simulink model "HybridPowertrain_TestBench_Final"  (R2017a)
settings: Solver=ode1  StartTime=0.0  StopTime=1400  FixedStep=0.01  RelTol=1e-3  EnableMultiTasking=on
undefined symbols (not defined in the file): AccActPos, air, Atm_temp, bms_inletair_temp, BMS_IstStrom, bms_maxchargecurrent, bms_maxdischargecurrent, BMS_Notfallkuehlung, BMS_SOC, BrkPdlPos, cal, Cells, Chg, D1_Commanded_Torque, D1_DC_Bus_Voltage, D2_Motor_Speed, D2_Torque_Feedback, DriverControls, EcoCAR3_Lib, Em, EngActStdyStTorq, Engine, EngSpd, env, ESS, fd, g, gb, Gearbox, GearBox, gps_lat, gps_long, Grade, I_loss, IMG, InstFuelConsmpRate, KeyPosition, lib_ESS_plant_V1_2, Loss, max_vehicle_rad_air_flow, mot, mph2kph, mph2ms, NeutralGear, ParkGear, PPEI_Engine_General_Status_2__ThrPos, PTEI_Engine_Torque_Status__EngActStdyStTorq, R_0, R_1, Ratio, RegenBrkDisable, rho, SampleTime, ShiftLeverPosition, SOC_bp, SOC_init, Spd, Speed, SW_CS_ON, SW_Engine_ON ... (+15)
libraries: simulink x39, fl_lib x13, nesl_utility x8, Utility x1, EC2_libraries x1
(part 2 of 5)

== system HybridPowertrain_TestBench_Final/ESS/ESS ==
  note: Sensors
  note: Discharge is Negative!
  note: $Author: eo1000 $
      | $Rev: 431 $
      | $Date: 2016-09-24 14:28:33 -0500 (Sat, 24 Sep 2016) $
  "In " : Inport
  "Crr " : Inport  Port=2
  0 current : Memory  InheritSampleTime=on
  Bosch_Li_Cell : Subsystem
  Bus Creator1 : BusCreator  Inputs=5
  Constant{1..4} (4 alike) : Constant  Value=0
  Cooling_Loop : Subsystem
  Cooling_Loop1 : Subsystem  Commented=on
  Data Type Conversion : DataTypeConversion  OutDataTypeStr=double
  Fault_Insertion : Subsystem
  Gain1 : Gain  Gain=Cells*0.9824
  Rate Transition : RateTransition  X0=273.15+25
  Switch1 : Switch  Threshold=1
  Switch2 : Switch  Threshold=1
  Switch3 : Switch  Threshold=5
  Switch4 : Switch  Threshold=5
  To Workspace1 : ToWorkspace  VariableName=SOC  SampleTime=-1
      settings: Decimation=WORKSPACE_DECIMATION
  To Workspace4 : ToWorkspace  VariableName=ess_current_hist  SampleTime=-1
      settings: Decimation=WORKSPACE_DECIMATION
  To Workspace5 : ToWorkspace  VariableName=ess_term_voltage_hist  SampleTime=-1
      settings: Decimation=WORKSPACE_DECIMATION
  To Workspace6 : ToWorkspace  VariableName=ess_mainc_hist  SampleTime=-1
      settings: Decimation=WORKSPACE_DECIMATION
  tloop2 : Gain  Gain=-1
  out : Outport
  Voltage : Outport  Port=2
  tag scope: SOC=global, ess_temp=global
  wires:
  "In "/1 -> [ess_mainc_stat]
  Bus Creator1/1 -> out/1
  Data Type Conversion/1 -> To Workspace6/1
  Constant2/1 -> Switch1/3
  Switch1/1 -> To Workspace4/1  "ess_ibat"
  Gain1/1 -> Switch2/1  "output voltage"
  [ess_mainc_stat] -> Switch3/2, Data Type Conversion/1, Switch3/3  "MainC"
  Constant3/1 -> Switch2/3
  Switch2/1 -> Bus Creator1/1, Voltage/1, To Workspace5/1  "ess_vbat"
  [SOC] -> Bus Creator1/5  "ess_soc"
  Bosch_Li_Cell/1(V) -> Bus Creator1/3, Gain1/1  "Vcell"
  Constant1/1 -> Switch3/1
  Switch3/1 -> Switch1/2
  [ess_mainc_stat] -> Switch4/3, Switch4/2  "MainC"
  Constant4/1 -> Switch4/1
  Switch4/1 -> Switch2/2
  0 current/1 -> tloop2/1, Bus Creator1/4, Switch1/1  "ess_ibat"
  "Crr "/1 -> 0 current/1  "current"
  Bosch_Li_Cell/3(T) -> Rate Transition/1  "T"
  Bosch_Li_Cell/2(SOC) -> To Workspace1/1, [SOC]  "SOC"
  tloop2/1 -> Bosch_Li_Cell/1(I)
  Fault_Insertion/1(Out1) -> Bus Creator1/2, [ess_temp]
  Rate Transition/1 -> Fault_Insertion/1(In1)
  connections:
  Cooling_Loop/RConn1 -- Bosch_Li_Cell/LConn1

== system HybridPowertrain_TestBench_Final/ESS/Inputs ==
  Bus Creator1 : BusCreator  Inputs=2
  CAN_fromHCU : Subsystem
  Digital_fromHCU : Subsystem
  Inputs : Outport
  wires:
  Digital_fromHCU/1(Outputs) -> Bus Creator1/2  "Digital"
  CAN_fromHCU/1(Outputs) -> Bus Creator1/1  "CAN"
  Bus Creator1/1 -> Inputs/1

== system HybridPowertrain_TestBench_Final/ESS/Outputs ==
  Outputs : Inport
  tag scope: BMS_to_HCU=global
  wires:
  Outputs/1 -> [BMS_to_HCU]  "BMS_CAN"

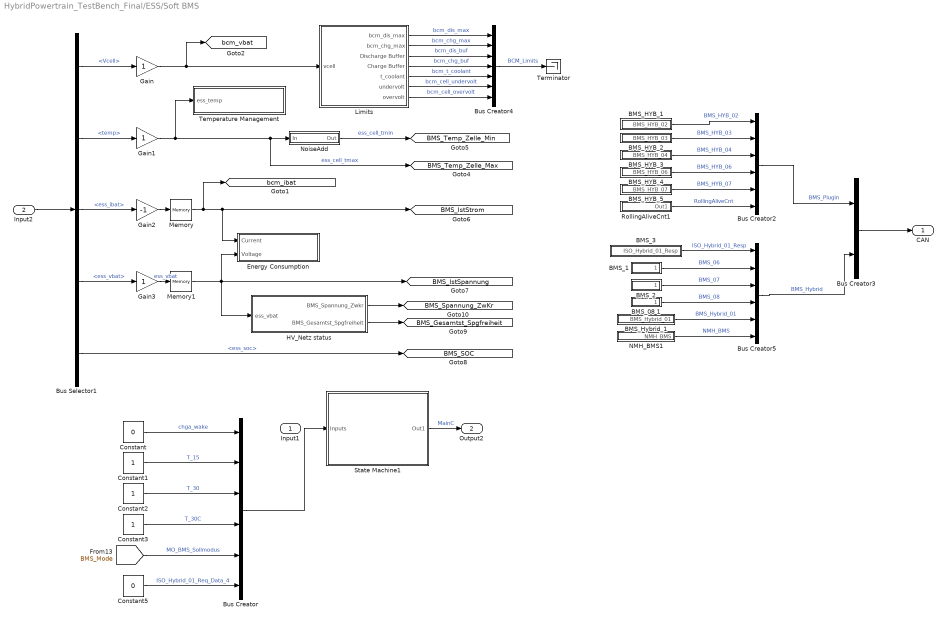
== system HybridPowertrain_TestBench_Final/ESS/Soft BMS ==
  Input1 : Inport
  Input2 : Inport  Port=2
  BMS_08 1 : Subsystem
  BMS_1 : Subsystem
  BMS_2 : Subsystem
  BMS_3 : Subsystem
  BMS_HYB_1 : Subsystem
  BMS_HYB_2 : Subsystem
  BMS_HYB_3 : Subsystem
  BMS_HYB_4 : Subsystem
  BMS_HYB_5 : Subsystem
  BMS_Hybrid_1 : Subsystem
  Bus Creator : BusCreator  Inputs=6
  Bus Creator2 : BusCreator  Inputs=6
  Bus Creator3 : BusCreator  Inputs=2
  Bus Creator4 : BusCreator  Inputs=7
  Bus Creator5 : BusCreator  Inputs=6
  Bus Selector1 : BusSelector  OutputSignals=Vcell,temp,ess_ibat,ess_vbat,ess_soc
  Constant : Constant  Value=0
  Constant1 : Constant
  Constant2 : Constant
  Constant3 : Constant
  Constant5 : Constant  Value=0
  Energy Consumption : Subsystem
  Gain : Gain
  Gain1 : Gain
  Gain2 : Gain  Gain=-1
  Gain3 : Gain
  HV_Netz status : Subsystem
  Limits : Subsystem
  Memory : Memory
  Memory1 : Memory
  NMH_BMS1 : Subsystem
  NoiseAdd : Subsystem
  RollingAliveCnt1 : Subsystem
  State Machine1 : Subsystem
  Temperature Management : Subsystem
  Terminator : Terminator
  CAN : Outport
  Output2 : Outport  Port=2
  tag scope: BMS_Gesamtst_Spgfreiheit=global, BMS_IstSpannung=global, BMS_IstStrom=global, BMS_SOC=global, BMS_Spannung_ZwKr=global, BMS_Temp_Zelle_Max=global, BMS_Temp_Zelle_Min=global, bcm_ibat=global, bcm_vbat=global
  wires:
  State Machine1/1(Out1) -> Output2/1  "MainC"
  Gain3/1 -> Memory1/1  "ess_vbat"
  Gain2/1 -> Memory/1
  Gain/1 -> [bcm_vbat], Limits/1(vcell)
  Bus Creator/1 -> State Machine1/1(Inputs)
  Input2/1 -> Bus Selector1/1
  Bus Selector1/3 -> Gain2/1  "<ess_ibat>"
  NoiseAdd/1(Out) -> [BMS_Temp_Zelle_Min]  "ess_cell_tmin"
  Bus Selector1/1 -> Gain/1  "<Vcell>"
  Bus Selector1/2 -> Gain1/1  "<temp>"
  Gain1/1 -> Temperature Management/1(ess_temp), NoiseAdd/1(In), [BMS_Temp_Zelle_Max]  "ess_cell_tmax"
  Limits/1(bcm_dis_max) -> Bus Creator4/1  "bcm_dis_max"
  Limits/3(Discharge Buffer) -> Bus Creator4/3  "bcm_dis_buf"
  Limits/4(Charge Buffer) -> Bus Creator4/4  "bcm_chg_buf"
  Limits/5(t_coolant) -> Bus Creator4/5  "bcm_t_coolant"
  Limits/2(bcm_chg_max) -> Bus Creator4/2  "bcm_chg_max"
  Bus Creator4/1 -> Terminator/1  "BCM_Limits"
  Bus Selector1/5 -> [BMS_SOC]  "<ess_soc>"
  Bus Selector1/4 -> Gain3/1  "<ess_vbat>"
  Limits/6(undervolt) -> Bus Creator4/6  "bcm_cell_undervolt"
  Limits/7(overvolt) -> Bus Creator4/7  "bcm_cell_overvolt"
  Bus Creator3/1 -> CAN/1
  HV_Netz status/1(BMS_Spannung_Zwkr) -> [BMS_Spannung_ZwKr]
  HV_Netz status/2(BMS_Gesamtst_Spgfreiheit) -> [BMS_Gesamtst_Spgfreiheit]
  Memory/1 -> [bcm_ibat], Energy Consumption/1(Current), [BMS_IstStrom]
  Memory1/1 -> [BMS_IstSpannung], HV_Netz status/1(ess_vbat), Energy Consumption/2(Voltage)
  NMH_BMS1/1(NMH_BMS) -> Bus Creator5/6  "NMH_BMS"
  BMS_HYB_2/1(BMS_HYB_03) -> Bus Creator2/2  "BMS_HYB_03"
  BMS_HYB_5/1(BMS_HYB_07) -> Bus Creator2/5  "BMS_HYB_07"
  BMS_Hybrid_1/1(BMS_Hybrid_01) -> Bus Creator5/5  "BMS_Hybrid_01"
  BMS_2/1(BMS_07) -> Bus Creator5/3  "BMS_07"
  BMS_HYB_3/1(BMS_HYB_04) -> Bus Creator2/3  "BMS_HYB_04"
  BMS_HYB_1/1(BMS_HYB_02) -> Bus Creator2/1  "BMS_HYB_02"
  BMS_HYB_4/1(BMS_HYB_06) -> Bus Creator2/4  "BMS_HYB_06"
  BMS_1/1(BMS_06) -> Bus Creator5/2  "BMS_06"
  BMS_08 1/1(BMS_08) -> Bus Creator5/4  "BMS_08"
  Bus Creator5/1 -> Bus Creator3/2  "BMS_Hybrid"
  Bus Creator2/1 -> Bus Creator3/1  "BMS_Plugin"
  BMS_3/1(ISO_Hybrid_01_Resp) -> Bus Creator5/1  "ISO_Hybrid_01_Resp"
  RollingAliveCnt1/1(Out1) -> Bus Creator2/6  "RollingAliveCnt"
  Constant/1 -> Bus Creator/1  "chga_wake"
  Constant1/1 -> Bus Creator/2  "T_15"
  Constant3/1 -> Bus Creator/4  "T_30C"
  Constant2/1 -> Bus Creator/3  "T_30"
  [BMS_Mode] -> Bus Creator/5  "MO_BMS_Sollmodus"
  Constant5/1 -> Bus Creator/6  "ISO_Hybrid_01_Req_Data_4"

== system HybridPowertrain_TestBench_Final/ICE Simple/Engine Plant Modified ==
  "In " : Inport
  eng_spd_out : Inport  Port=2
  Core Engine : Subsystem
      mask Display: image(imread('EngineShortBlock.jpg'),'center')
  ECU Actuators : Subsystem
  ECU Sensors : Subsystem
  Fuel Supply : Subsystem
      mask Display: image(imread('FuelTank.jpg'),'center')
  Radiator : Subsystem  Commented=on  AncestorBlock=lib_Vehicle/Vehicle_Plant_Model/Radiator
  Out : Outport
  eng_shaft_out : Outport  Port=2
  tag scope: EngCrankCmd=global, EngRunAtv=global, EngShutdown=global, Eng_Fan=global, Eng_Temp=global, FuelPumpEnable=global, ThrPstCmd_pct=global, VehSpdAvgDrvn_Eng=global
  wires:
  ECU Actuators/5(Out5) -> [EngShutdown]
  [FuelLevelPct] -> ECU Sensors/4(In4)  "FuelLevelPct"
  [EmsHC] -> ECU Sensors/6(In6)  "HC_g/s"
  [EngPe] -> ECU Sensors/5(In5)  "PE_0_1"
  [EmsCO] -> ECU Sensors/7(In7)  "CO_g/s"
  [EmsCO2] -> ECU Sensors/8(In8)  "CO2_g/s"
  [EmsNOx] -> ECU Sensors/9(In9)  "NOx_g/s"
  Fuel Supply/1(Available Fuel) -> Core Engine/2(Available Fuel)
  ECU Actuators/4(Out4) -> [FuelPumpEnable]
  ECU Actuators/1(Out1) -> [ThrPstCmd_pct]
  "In "/1 -> ECU Actuators/1(In1)
  [EngBrkTrq] -> ECU Sensors/1(In1)  "EngActStdyStTorq_Nm"
  [AdvFuelFlowEst] -> ECU Sensors/3(In3)  "EngFuelFlow_g/s"
  [EngSpd_RPM] -> ECU Sensors/2(In2)  "EngSpd_RPM"
  ECU Actuators/2(Out2) -> [EngCrankCmd]
  ECU Actuators/3(Out3) -> [EngRunAtv]
  Core Engine/1(eng_shaft_out) -> eng_shaft_out/1
  eng_spd_out/1 -> Core Engine/1(Engine Speed (rad/s))
  [EngTemp] -> ECU Sensors/10(In10)  "Eng_Temp"
  [Eng_Fan] -> Radiator/2(Fans)
  [Eng_Temp] -> Radiator/1(EngCltTmp)
  ECU Actuators/6(Out6) -> [Eng_Temp]
  ECU Actuators/7(Out7) -> [Eng_Fan]
  ECU Actuators/8(Out8) -> [VehSpdAvgDrvn_Eng]
  ECU Sensors/1(Out1) -> Out/1

== system HybridPowertrain_TestBench_Final/ICE Simple/Inputs ==
  Analog : Subsystem
  Bus Creator : BusCreator  Inputs=2
  CAN_from_HCU : Subsystem
  Inputs : Outport
  wires:
  CAN_from_HCU/1(Out1) -> Bus Creator/1  "CAN"
  Analog/1(Out1) -> Bus Creator/2  "Analog"
  Bus Creator/1 -> Inputs/1

== system HybridPowertrain_TestBench_Final/ICE Simple/Soft ECM ==
  note: Should check lookup table with GM
  In : Inport
  In1 : Inport  Port=2
  Bus Creator1 : BusCreator  Inputs=3
  Bus Creator2 : BusCreator  Inputs=9
  Bus Selector : BusSelector  OutputSignals=EngSpd_RPM
  Bus Selector1 : BusSelector  Commented=on  OutputSignals=Analog.EngAppReq,CAN.to EBCAN.ISO_Hybrid_01_Req.ISO_Hybrid_01_Req_Data_4,CAN.to EBCAN.PPEI_Trans_General_Status_2.TrnsShftLvrPos
  Bus Selector2 : BusSelector  OutputSignals=Eng_Temp,EngFuelFlow_g/s
  Bus Selector3 : BusSelector  OutputSignals=drv_APP1,KeyPos,ShiftLvrPos
  Data Type Conversion : DataTypeConversion  OutDataTypeStr=int8
  Data Type Conversion1 : DataTypeConversion  OutDataTypeStr=int8
  ECM_RollingAliveCnt : Subsystem
  Fuel Consumption : Subsystem
  Logic : Stateflow chart  TreatAsAtomicUnit=on
  Memory1 : Memory  X0=Engine.Init_T_amb
  Memory2 : Memory  InheritSampleTime=on
  temp vs fan : Lookup_n-D  NumberOfTableDimensions=1  BreakpointsForDimension1=[0:1:100]  Table=[0:0.01:1]  InternalRulePriority=Speed  RndMeth=Simplest  InputSameDT=on
  Out : Outport
  Out1 : Outport  Port=2
  wires:
  Logic/3(EngRunAtv) -> Bus Creator2/3  "EngRunAtv"
  Bus Selector/1 -> Logic/4(EngSpd_RPM)  "<EngSpd_RPM>"
  Bus Selector3/1 -> Memory2/1  "<drv_APP1>"
  Logic/2(EngCrankCmd) -> Bus Creator2/2  "Eng12vStrtrMtrCmmdOn"
  Bus Creator1/1 -> Out/1  "ECM_CAN"
  Bus Creator2/1 -> Out1/1, Bus Creator1/1  "ECM_to_Actuators"
  Logic/1(ThrottleCmd) -> Bus Creator2/1  "ThrPosCmd_%"
  In1/1 -> Bus Selector2/1, Bus Creator1/3, Bus Selector/1  "Sensors_to_ECM"
  In/1 -> Bus Selector1/1  "HCU_to_ECM"
  Logic/4(FuelPumpEnable) -> Bus Creator2/4  "FuelPumpEnable"
  Bus Selector3/2 -> Data Type Conversion/1  "<KeyPos>"
  [VehSpdAvgDrvn] -> Bus Creator2/6, Logic/5(VehSpdAvgDrvn)  "VehSpdAvgDrvn"
  Bus Selector3/3 -> Data Type Conversion1/1  "<ShiftLvrPos>"
  Logic/5(EngShutdown) -> Bus Creator2/5  "EngShutdown"
  Bus Selector2/1 -> Memory1/1, temp vs fan/1  "<Eng_Temp>"
  Bus Selector2/2 -> Fuel Consumption/1(Fuel Consumption)  "<EngFuelFlow_g/s>"
  Fuel Consumption/1(fuel consumption) -> Bus Creator1/2  "Eng_fuel_consumption"
  temp vs fan/1 -> Bus Creator2/9  "fan_cmd"
  Memory1/1 -> Bus Creator2/8  "Eng_Temp"
  Memory2/1 -> Logic/1(drvAPP)
  ECM_RollingAliveCnt/1(Out1) -> Bus Creator2/7
  Data Type Conversion/1 -> Logic/2(SysPwrMd)
  Data Type Conversion1/1 -> Logic/3(ShftLvrPos)
  [Driver_Request2] -> Bus Selector3/1

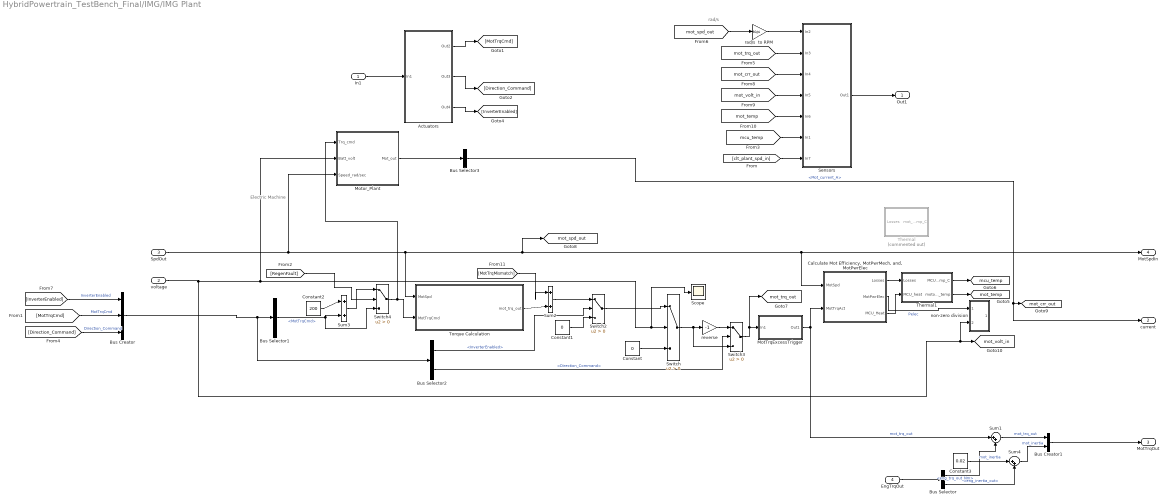
== system HybridPowertrain_TestBench_Final/IMG/IMG Plant ==
  note: Electric Machine
  note: rad/s
  "In1 " : Inport
  voltage : Inport  Port=2
  SpdOut : Inport  Port=3
  EngTrqOut : Inport  Port=4
  " Actuators" : Subsystem
  Bus Creator : BusCreator  Inputs=3
  Bus Creator1 : BusCreator  Inputs=2
  Bus Selector : BusSelector  OutputSignals=eng_trq_out_Nm,eng_inertia_out
  Bus Selector1 : BusSelector  OutputSignals=MotTrqCmd
  Bus Selector2 : BusSelector  OutputSignals=InverterEnabled,Direction_Command
  Bus Selector3 : BusSelector  OutputSignals=Mot_current_A
  "Calculate Mot Efficiency, MotPwrMech, and, MotPwrElec" : Subsystem
  Constant : Constant  Value=0
  Constant1 : Constant  Value=0
  Constant2 : Constant  Value=200
  Constant3 : Constant  Value=0.02
  MotTrqExcessTrigger : Subsystem
  Motor_Plant : Subsystem
  Scope : Scope
  Sensors : Subsystem
  Sum{1..4} (4 alike) : Sum  Inputs=|++
  Switch{,2..4} (4 alike) : Switch  Criteria=u2 > Threshold
  Thermal : Subsystem  Commented=on
  Thermal1 : Subsystem
  Torque Calculation : Subsystem
  non-zero division : Subsystem
      mask Display: disp('divider \n I1/I2')
  rad/s  to RPM : Gain  Gain=30/pi
  reverse : Gain  Gain=-1
  Out1 : Outport
  current : Outport  Port=2
  MotTrqOut : Outport  Port=3
  MotSpdIn : Outport  Port=4
  tag scope: mcu_temp=global, mot_crr_out=global, mot_spd_out=global, mot_temp=global, mot_trq_out=global, mot_volt_in=global
  wires:
  [mot_temp] -> Sensors/5(In6)
  [mot_crr_out] -> Sensors/3(In4)
  "In1 "/1 -> " Actuators"/1(In1)
  [mot_volt_in] -> Sensors/4(In5)
  " Actuators"/1(Out2) -> [MotTrqCmd]
  Sensors/1(Out1) -> Out1/1
  [mot_trq_out] -> Sensors/2(In3)
  SpdOut/1 -> Motor_Plant/3(Speed_rad/sec), Torque Calculation/1(MotSpd), [mot_spd_out], MotSpdIn/1, "Calculate Mot Efficiency, MotPwrMech, and, MotPwrElec"/1(MotSpd)
  Bus Selector3/1 -> current/1, [mot_crr_out]  "<Mot_current_A>"
  [mcu_temp] -> Sensors/6(In1)
  [clt_plant_spd_in] -> Sensors/7(In7)
  " Actuators"/2(Out3) -> [Direction_Command]
  " Actuators"/3(Out4) -> [InverterEnabled]
  [Direction_Command] -> Bus Creator/3  "Direction_Command"
  [InverterEnabled] -> Bus Creator/1  "InverterEnabled"
  [MotTrqCmd] -> Bus Creator/2  "MotTrqCmd"
  [mot_spd_out] -> rad/s  to RPM/1
  rad/s  to RPM/1 -> Sensors/1(In2)
  Thermal1/1(MCU_temp_C) -> [mcu_temp]
  Constant2/1 -> Sum3/1
  Switch4/1 -> Motor_Plant/1(Trq_cmd), Torque Calculation/2(MotTrqCmd)
  Sum3/1 -> Switch4/1
  [RegenFault] -> Switch4/2
  Switch3/1 -> [mot_trq_out], MotTrqExcessTrigger/1(In1)
  reverse/1 -> Switch3/1
  Bus Selector2/2 -> Switch3/2  "<Direction_Command>"
  Switch2/1 -> Switch/1
  Constant1/1 -> Switch2/3
  Bus Selector2/1 -> Switch2/2  "<InverterEnabled>"
  Bus Selector1/1 -> Switch4/3, Sum3/2  "<MotTrqCmd>"
  Bus Creator/1 -> Bus Selector2/1, Bus Selector1/1
  Sum2/1 -> Switch2/1
  Torque Calculation/1(mot_trq_out) -> Sum2/2
  [MotTrqMismatch] -> Sum2/1
  Switch/1 -> Switch3/3, reverse/1
  Thermal1/2(motor_temp) -> [mot_temp]
  "Calculate Mot Efficiency, MotPwrMech, and, MotPwrElec"/3(MCU_Heat) -> Thermal1/2(MCU_heat)
  Constant/1 -> Switch/3
  "Calculate Mot Efficiency, MotPwrMech, and, MotPwrElec"/1(Losses) -> Thermal1/1(Losses)
  MotTrqExcessTrigger/1(Out1) -> Sum1/1, "Calculate Mot Efficiency, MotPwrMech, and, MotPwrElec"/2(MotTrqAct)  "mot_trq_out"
  "Calculate Mot Efficiency, MotPwrMech, and, MotPwrElec"/2(MotPwrElec) -> non-zero division/1(In1)  "Pelec"
  voltage/1 -> non-zero division/2(In2), [mot_volt_in], Motor_Plant/2(Batt_volt), Scope/1, Switch/2
  Bus Creator1/1 -> MotTrqOut/1
  Sum4/1 -> Bus Creator1/2  "mot_inertia"
  EngTrqOut/1 -> Bus Selector/1
  Sum1/1 -> Bus Creator1/1  "mot_trq_out"
  Bus Selector/2 -> Sum4/2  "<eng_inertia_out>"
  Constant3/1 -> Sum4/1  "mot_inertia"
  Bus Selector/1 -> Sum1/2  "<eng_trq_out_Nm>"
  Motor_Plant/1(Mot_out) -> Bus Selector3/1

== system HybridPowertrain_TestBench_Final/IMG/Soft MCU ==
  In : Inport
  In1 : Inport  Port=2
  Bus Creator : BusCreator  Inputs=6
  Bus Creator1 : BusCreator  Inputs=2
  Bus Selector : BusSelector  OutputSignals=mot_spd_out,mot_trq_out
  Bus Selector1 : BusSelector  Commented=on  OutputSignals=M192_Command_Message.Inverter_Enable,M192_Command_Message.Torque_Command
  Constant : Constant  Value=0
  Constant1 : Constant
  Data Type Conversion{1..4} (4 alike) : DataTypeConversion
  ForwardDirection : Constant  Value=0
  MCU_CAN_rolling : Subsystem
  Memory : Memory
  Scope : Scope  NumInputPorts=5
  Switch : Switch  Threshold=1
  Torque Calculation : Subsystem
  Out : Outport
  Out1 : Outport  Port=2
  wires:
  In1/1 -> Bus Creator1/2, Bus Selector/1  "Sensors_to_MCU"
  Bus Creator1/1 -> Out/1  "MCU_CAN"
  In/1 -> Bus Selector1/1  "HCU_to_MCU"
  [MotTrqCmd] -> Torque Calculation/1(MotTrqReq), Scope/2, Data Type Conversion4/1
  Bus Creator/1 -> Bus Creator1/1, Out1/1  "MCU_to _Actuator"
  Constant1/1 -> Memory/1, Switch/2, Scope/3
  Constant/1 -> Switch/3
  Bus Selector/1 -> Scope/5, Torque Calculation/2(MotSpd)  "<mot_spd_out>"
  Torque Calculation/1(mot_trq_out) -> Switch/1
  Data Type Conversion1/1 -> Bus Creator/3  "InverterEnabled"
  Bus Selector/2 -> Scope/4, Torque Calculation/3(MotTrqFdbck), Data Type Conversion2/1  "<mot_trq_out>"
  Data Type Conversion2/1 -> Bus Creator/4  "MotTrqFdbck"
  Memory/1 -> Data Type Conversion1/1
  Switch/1 -> Data Type Conversion3/1  "MotTrqCmd"
  Data Type Conversion3/1 -> Bus Creator/2, Scope/1  "MotTrqCmd"
  Data Type Conversion4/1 -> Bus Creator/1  "Torque_Command"
  MCU_CAN_rolling/1(Out1) -> Bus Creator/5  "D3_Power_On_Timer"
  ForwardDirection/1 -> Bus Creator/6  "Direction_Command"

== system HybridPowertrain_TestBench_Final/Measurements_hybrid/DriverControls1 ==
  cmd : Inport
  meas : Inport  Port=2
  BrakeForce : Gain  Gain=100
  Memory : Memory
  Memory1 : Memory
  PID Controller : simulink/Continuous/PID Controller  Controller=PI  TimeDomain=Continuous-time  SampleTime=-1  IntegratorMethod=Forward Euler  FilterMethod=Forward Euler  Form=Parallel  UseFilter=on  ControllerParametersSource=internal  P=0.1  I=0.001  D=0  N=100  InitialConditionSource=internal  InitialConditionForIntegrator=0  InitialConditionForFilter=0  ExternalReset=none  LimitOutput=off  UpperSaturationLimit=1  LowerSaturationLimit=0  LinearizeAsGain=on  AntiWindupMode=clamping  Kb=1  TrackingMode=off  Kt=1  PParamMin=[]  PParamMax=[]  IParamMin=[]  IParamMax=[]  DParamMin=[]  DParamMax=[]  NParamMin=[]  NParamMax=[]  KbParamMin=[]  KbParamMax=[]  KtParamMin=[]  KtParamMax=[]  POutMin=[]  POutMax=[]  IOutMin=[]  IOutMax=[]  DOutMin=[]  DOutMax=[]  NOutMin=[]  NOutMax=[]  KbOutMin=[]  KbOutMax=[]  KtOutMin=[]  KtOutMax=[]  IntegratorOutMin=[]  IntegratorOutMax=[]  FilterOutMin=[]  FilterOutMax=[]  SumOutMin=[]  SumOutMax=[]  SumI1OutMin=[]  SumI1OutMax=[]  SumI2OutMin=[]  SumI2OutMax=[]  SumI3OutMin=[]  SumI3OutMax=[]  SumDOutMin=[]  SumDOutMax=[]  SaturationOutMin=[]  SaturationOutMax=[]  IntegratorContinuousStateAttributes=''  IntegratorStateMustResolveToSignalObject=off  IntegratorRTWStateStorageClass=Auto  FilterContinuousStateAttributes=''  FilterStateMustResolveToSignalObject=off  FilterRTWStateStorageClass=Auto  DifferentiatorICPrevScaledInput=0  DifferentiatorOutMin=[]  DifferentiatorOutMax=[]  InitialConditionSetting=State (most efficient)
  PID Controller1 : simulink/Continuous/PID Controller  Controller=PI  TimeDomain=Continuous-time  SampleTime=-1  IntegratorMethod=Forward Euler  FilterMethod=Forward Euler  Form=Parallel  UseFilter=on  ControllerParametersSource=internal  P=0.1  I=0.001  D=0  N=100  InitialConditionSource=internal  InitialConditionForIntegrator=0  InitialConditionForFilter=0  ExternalReset=none  LimitOutput=on  UpperSaturationLimit=1  LowerSaturationLimit=-1  LinearizeAsGain=on  AntiWindupMode=clamping  Kb=1  TrackingMode=off  Kt=1  PParamMin=[]  PParamMax=[]  IParamMin=[]  IParamMax=[]  DParamMin=[]  DParamMax=[]  NParamMin=[]  NParamMax=[]  KbParamMin=[]  KbParamMax=[]  KtParamMin=[]  KtParamMax=[]  POutMin=[]  POutMax=[]  IOutMin=[]  IOutMax=[]  DOutMin=[]  DOutMax=[]  NOutMin=[]  NOutMax=[]  KbOutMin=[]  KbOutMax=[]  KtOutMin=[]  KtOutMax=[]  IntegratorOutMin=[]  IntegratorOutMax=[]  FilterOutMin=[]  FilterOutMax=[]  SumOutMin=[]  SumOutMax=[]  SumI1OutMin=[]  SumI1OutMax=[]  SumI2OutMin=[]  SumI2OutMax=[]  SumI3OutMin=[]  SumI3OutMax=[]  SumDOutMin=[]  SumDOutMax=[]  SaturationOutMin=[]  SaturationOutMax=[]  IntegratorContinuousStateAttributes=''  IntegratorStateMustResolveToSignalObject=off  IntegratorRTWStateStorageClass=Auto  FilterContinuousStateAttributes=''  FilterStateMustResolveToSignalObject=off  FilterRTWStateStorageClass=Auto  DifferentiatorICPrevScaledInput=0  DifferentiatorOutMin=[]  DifferentiatorOutMax=[]  InitialConditionSetting=State (most efficient)
  Pct : Gain  Gain=100
  Saturation1 : Saturate  UpperLimit=100  LowerLimit=0
  Saturation2 : Saturate  UpperLimit=100  LowerLimit=0
  Sum : Sum  Inputs=|+-
  Sum1 : Sum  Inputs=+-|
  brake : Outport
  throttle : Outport  Port=2
  wires:
  cmd/1 -> Sum/1, Sum1/2
  Sum1/1 -> PID Controller/1
  meas/1 -> Sum1/1, Sum/2
  PID Controller/1 -> BrakeForce/1
  Saturation1/1 -> Memory/1
  BrakeForce/1 -> Saturation1/1
  PID Controller1/1 -> Pct/1
  Memory/1 -> brake/1
  Sum/1 -> PID Controller1/1
  Pct/1 -> Saturation2/1
  Saturation2/1 -> Memory1/1
  Memory1/1 -> throttle/1

== system HybridPowertrain_TestBench_Final/Measurements_hybrid/Subsystem ==
  In1 : Inport
  Add1 : Sum  Inputs=+++
  Add2 : Sum
  Constant1 : Constant  Value=0
  Constant2 : Constant  Value=cal.APP.Mismatch_Value+0.1
  Constant3 : Constant  Value=0
  Constant4 : Constant  Value=cal.APP2.IN_Max_SC_Prcnt+1
  Constant5 : Constant  Value=0
  Constant6 : Constant  Value=cal.APP2.IN_Max_SC_Prcnt+1
  Switch : Switch  Threshold=1
  Switch1 : Switch  Threshold=1
  Switch2 : Switch  Threshold=1
  APP1 : Outport
  APP2 : Outport  Port=2
  wires:
  Switch2/1 -> Add2/2
  Add2/1 -> APP1/1  "drv_APP1"
  [APP2_OOR_ON] -> Switch2/2
  Constant6/1 -> Switch2/1
  Constant5/1 -> Switch2/3
  In1/1 -> Add1/1, Add2/1
  Add1/1 -> APP2/1  "drv_APP2"
  Switch1/1 -> Add1/3
  [APP2_OOR_ON] -> Switch1/2
  Constant4/1 -> Switch1/1
  Constant3/1 -> Switch1/3
  Constant2/1 -> Switch/1
  Constant1/1 -> Switch/3
  Switch/1 -> Add1/2
  [Mismatch_APP_ON] -> Switch/2

== system HybridPowertrain_TestBench_Final/Measurements_stock/DriverControls ==
  cmd : Inport
  meas : Inport  Port=2
  Abs : Abs
  BrakeForce : Gain  Commented=on  Gain=100
  Clamping circuit : Subsystem  Commented=on
  Compare To Constant : simulink/Logic and Bit Operations/Compare To Constant  relop=>  const=10  OutDataTypeStr=boolean
  Compare To Constant1 : simulink/Logic and Bit Operations/Compare To Constant  relop=>  const=0  OutDataTypeStr=boolean
  Compare To Constant2 : simulink/Logic and Bit Operations/Compare To Constant  relop=<=  const=0  OutDataTypeStr=boolean
  Constant : Constant  Value=11.5
  Constant1 : Constant  Commented=on  DisableCoverage=on  Value=0  OutDataTypeStr=Inherit: Inherit via back propagation  PreserveConstantTs=on
  Constant2 : Constant  Value=0
  Constant3 : Constant  Value=0
  IntegralGain : Gain  Commented=on  Gain=0.001
  Integrator : Integrator  Commented=on
  Memory : Memory  Commented=on
  MinMax : MinMax  Function=max  Inputs=2
  PID Controller : simulink/Continuous/PID Controller  Commented=on  Controller=PI  TimeDomain=Continuous-time  SampleTime=-1  IntegratorMethod=Forward Euler  FilterMethod=Forward Euler  Form=Parallel  UseFilter=on  ControllerParametersSource=internal  P=0.1  I=0.001  D=0  N=100  InitialConditionSource=internal  InitialConditionForIntegrator=0  InitialConditionForFilter=0  ExternalReset=none  LimitOutput=off  UpperSaturationLimit=1  LowerSaturationLimit=0  LinearizeAsGain=on  AntiWindupMode=clamping  Kb=1  TrackingMode=off  Kt=1  PParamMin=[]  PParamMax=[]  IParamMin=[]  IParamMax=[]  DParamMin=[]  DParamMax=[]  NParamMin=[]  NParamMax=[]  KbParamMin=[]  KbParamMax=[]  KtParamMin=[]  KtParamMax=[]  POutMin=[]  POutMax=[]  IOutMin=[]  IOutMax=[]  DOutMin=[]  DOutMax=[]  NOutMin=[]  NOutMax=[]  KbOutMin=[]  KbOutMax=[]  KtOutMin=[]  KtOutMax=[]  IntegratorOutMin=[]  IntegratorOutMax=[]  FilterOutMin=[]  FilterOutMax=[]  SumOutMin=[]  SumOutMax=[]  SumI1OutMin=[]  SumI1OutMax=[]  SumI2OutMin=[]  SumI2OutMax=[]  SumI3OutMin=[]  SumI3OutMax=[]  SumDOutMin=[]  SumDOutMax=[]  SaturationOutMin=[]  SaturationOutMax=[]  IntegratorContinuousStateAttributes=''  IntegratorStateMustResolveToSignalObject=off  IntegratorRTWStateStorageClass=Auto  FilterContinuousStateAttributes=''  FilterStateMustResolveToSignalObject=off  FilterRTWStateStorageClass=Auto  DifferentiatorICPrevScaledInput=0  DifferentiatorOutMin=[]  DifferentiatorOutMax=[]
  PID Controller1 : simulink/Continuous/PID Controller  Controller=PI  TimeDomain=Continuous-time  SampleTime=-1  IntegratorMethod=Forward Euler  FilterMethod=Forward Euler  Form=Parallel  UseFilter=on  ControllerParametersSource=internal  P=0.1  I=0.001  D=0  N=100  InitialConditionSource=internal  InitialConditionForIntegrator=0  InitialConditionForFilter=0  ExternalReset=none  LimitOutput=on  UpperSaturationLimit=1  LowerSaturationLimit=-1  LinearizeAsGain=on  AntiWindupMode=clamping  Kb=1  TrackingMode=off  Kt=1  PParamMin=[]  PParamMax=[]  IParamMin=[]  IParamMax=[]  DParamMin=[]  DParamMax=[]  NParamMin=[]  NParamMax=[]  KbParamMin=[]  KbParamMax=[]  KtParamMin=[]  KtParamMax=[]  POutMin=[]  POutMax=[]  IOutMin=[]  IOutMax=[]  DOutMin=[]  DOutMax=[]  NOutMin=[]  NOutMax=[]  KbOutMin=[]  KbOutMax=[]  KtOutMin=[]  KtOutMax=[]  IntegratorOutMin=[]  IntegratorOutMax=[]  FilterOutMin=[]  FilterOutMax=[]  SumOutMin=[]  SumOutMax=[]  SumI1OutMin=[]  SumI1OutMax=[]  SumI2OutMin=[]  SumI2OutMax=[]  SumI3OutMin=[]  SumI3OutMax=[]  SumDOutMin=[]  SumDOutMax=[]  SaturationOutMin=[]  SaturationOutMax=[]  IntegratorContinuousStateAttributes=''  IntegratorStateMustResolveToSignalObject=off  IntegratorRTWStateStorageClass=Auto  FilterContinuousStateAttributes=''  FilterStateMustResolveToSignalObject=off  FilterRTWStateStorageClass=Auto  DifferentiatorICPrevScaledInput=0  DifferentiatorOutMin=[]  DifferentiatorOutMax=[]
  Pct : Gain  Gain=100
  ProportionalGain : Gain  Commented=on  Gain=0.1
  Saturation : Saturate  UpperLimit=100  LowerLimit=-100  LinearizeAsGain=off
  Saturation1 : Saturate  Commented=on  UpperLimit=100  LowerLimit=0
  Sum : Sum  Inputs=|+-
  Sum1 : Sum  Commented=on  Inputs=+-|
  Sum3 : Sum  Commented=on  Inputs=++|
  Switch : Switch  Criteria=u2 > Threshold
  Switch1 : Switch  Commented=on  Criteria=u2 > Threshold  SampleTime=SampleTime  InputSameDT=on
  Switch2 : Switch  Criteria=u2 > Threshold
  Switch3 : Switch  Criteria=u2 > Threshold
  brake : Outport
  throttle : Outport  Port=2
  wires:
  cmd/1 -> Compare To Constant/1, Sum/1, Sum1/2
  Sum1/1 -> PID Controller/1
  meas/1 -> Sum1/1, Sum/2
  PID Controller/1 -> BrakeForce/1
  Saturation1/1 -> Memory/1
  BrakeForce/1 -> Saturation1/1
  PID Controller1/1 -> Pct/1
  Memory/1 -> ?
  Compare To Constant/1 -> Switch/2
  MinMax/1 -> Switch/3
  Constant/1 -> MinMax/2
  Saturation/1 -> ?
  Sum/1 -> PID Controller1/1, ProportionalGain/1, IntegralGain/1
  Integrator/1 -> Sum3/2
  ProportionalGain/1 -> Sum3/1
  Sum3/1 -> Clamping circuit/1(preSat)
  Constant1/1 -> Switch1/1
  Clamping circuit/1(Clamp) -> Switch1/2
  IntegralGain/1 -> Integrator/1, Clamping circuit/2(preIntegrator), Switch1/3
  Compare To Constant1/1 -> Switch2/2
  Constant2/1 -> Switch2/3
  Switch2/1 -> throttle/1
  Pct/1 -> Compare To Constant2/1, Abs/1, Switch2/1, Compare To Constant1/1, Saturation/1, Switch/1, MinMax/1
  Compare To Constant2/1 -> Switch3/2
  Constant3/1 -> Switch3/3
  Switch3/1 -> brake/1
  Abs/1 -> Switch3/1

== system HybridPowertrain_TestBench_Final/Measurements_stock/Subsystem ==
  In1 : Inport
  Add1 : Sum  Inputs=+++
  Add2 : Sum
  Constant1 : Constant  Value=0
  Constant2 : Constant  Value=cal.APP.Mismatch_Value+0.1
  Constant3 : Constant  Value=0
  Constant4 : Constant  Value=cal.APP2.IN_Max_SC_Prcnt+1
  Constant5 : Constant  Value=0
  Constant6 : Constant  Value=cal.APP2.IN_Max_SC_Prcnt+1
  Switch : Switch  Threshold=1
  Switch1 : Switch  Threshold=1
  Switch2 : Switch  Threshold=1
  APP1 : Outport
  APP2 : Outport  Port=2
  wires:
  [Mismatch_APP_ON] -> Switch/2
  Switch/1 -> Add1/2
  Constant1/1 -> Switch/3
  Constant2/1 -> Switch/1
  Constant3/1 -> Switch1/3
  Constant4/1 -> Switch1/1
  [APP2_OOR_ON] -> Switch1/2
  Switch1/1 -> Add1/3
  Add1/1 -> APP2/1  "drv_APP2"
  In1/1 -> Add2/1, Add1/1
  Constant5/1 -> Switch2/3
  Constant6/1 -> Switch2/1
  [APP2_OOR_ON] -> Switch2/2
  Add2/1 -> APP1/1  "drv_APP1"
  Switch2/1 -> Add2/2

== system HybridPowertrain_TestBench_Final/Transmission/Inputs ==
  Analog_fromHCU : Subsystem
  Bus Creator1 : BusCreator  Inputs=3
  CAN_fromHCU : Subsystem
  Digital_fromHCU : Subsystem
  Inputs : Outport
  wires:
  Digital_fromHCU/1(Outputs) -> Bus Creator1/2  "Digital"
  CAN_fromHCU/1(Outputs) -> Bus Creator1/1  "CAN"
  Bus Creator1/1 -> Inputs/1
  Analog_fromHCU/1(Outputs) -> Bus Creator1/3

== system HybridPowertrain_TestBench_Final/Transmission/Outputs ==
  Outputs : Inport
  tag scope: TCM_to_HCU=global
  wires:
  Outputs/1 -> [TCM_to_HCU]  "TCM_CAN"

== system HybridPowertrain_TestBench_Final/Transmission/Soft TCM ==
  In : Inport
  In1 : Inport  Port=2
  6L45 Logic : Stateflow chart  TreatAsAtomicUnit=on
  Bus Creator : BusCreator  Inputs=3
  Bus Creator1 : BusCreator  Inputs=2
  Bus Selector : BusSelector  OutputSignals=impeller_spd_rads,turbine_spd_rads
  Bus Selector1 : BusSelector  Commented=on  OutputSignals=CAN.PPEI_Engine_General_Status_1.AccActPos,CAN.PPEI_Vehicle_Speed_and_Distance.VehSpdAvgDrvn
  Bus Selector2 : BusSelector  OutputSignals=drv_APP1,Veh_Spd
  Data Type Conversion : DataTypeConversion
  TorqConv Lockup threshold : Constant  Value=tc.plant.init.lock_thresh
  Out : Outport
  Out1 : Outport  Port=2
  wires:
  TorqConv Lockup threshold/1 -> 6L45 Logic/1(tc_lockup_thrsh)
  6L45 Logic/1(TransEstGear) -> Bus Creator/1
  Data Type Conversion/1 -> Bus Creator/3, 6L45 Logic/7(ShftLvrPos)  "TrnsShftLvrPos"
  In1/1 -> Bus Selector/1, Bus Creator1/2  "Sensors_to_TCM"
  Bus Creator1/1 -> Out/1  "TCM_CAN"
  In/1 -> Bus Selector1/1  "HCU_to_TCM"
  Bus Selector/2 -> 6L45 Logic/5(tc_spd_out)  "<turbine_spd_rads>"
  Bus Selector/1 -> 6L45 Logic/4(tc_spd_in)  "<impeller_spd_rads>"
  [chas_plant_lin_spd_out] -> 6L45 Logic/3(VehicleSpeed)
  Bus Selector2/1 -> 6L45 Logic/2(drvAPP)  "<drv_APP1>"
  Bus Creator/1 -> Out1/1, Bus Creator1/1  "TCM_to _Actuator"
  6L45 Logic/2(LockupCmd) -> Bus Creator/2
  [drv_BPP_percent] -> 6L45 Logic/6(drvBPP)
  [ShftLvrPos] -> Data Type Conversion/1  "TrnsShftLvrPos"
  [Driver_Request2] -> Bus Selector2/1

== system HybridPowertrain_TestBench_Final/Transmission/Transmission Plant ==
  "In1 " : Inport
  TorqConvShaftIn : Inport  Port=2
  GearboxSpdOut : Inport  Port=3
  " Actuators" : Subsystem
  Gearbox : Subsystem
      mask Display:
      | image('Images\Gearbox.jpg')
      | color('red');
      | port_label('Input',1,'Gear');
      | port_label('Input',2,'ShftIn');
      | port_label('Input',3,'SpdOut');
      | port_label('Output',1,'ShaftOut');
      | port_label('Output',2,'SpdIn');
  Sensors : Subsystem
  Torque Converter : Subsystem
      mask Display:
      | image('Images\TorqConv.jpg')
      | color('red');
      | port_label('Input',2,'ShaftIn');
      | port_label('Input',3,'SpdOut');
      | port_label('Output',1,'ShaftOut');
      | port_label('Output',2,'SpdIn');
  Out1 : Outport
  GearboxShaftOut : Outport  Port=2
  TorqConvSpdIn : Outport  Port=3
  tag scope: TransEstGear=global
  wires:
  Torque Converter/2(cpl_spd_in) -> TorqConvSpdIn/1
  Gearbox/2(gb_spd_in) -> Torque Converter/3(tc_spd_out)
  TorqConvShaftIn/1 -> Torque Converter/2(tc_shaft_in)
  Gearbox/1(gb_trq_out gb_inertia_out) -> GearboxShaftOut/1
  " Actuators"/1(Out2) -> [TransEstGear]
  [tc_trq_out] -> Sensors/4(In5)
  [gb_spd_out] -> Sensors/5(In6)
  [gb_trq_out] -> Sensors/6(In7)
  [tc_spd_out] -> Sensors/2(In3)
  [tc_spd_in] -> Sensors/1(In2)
  [tc_trq_in] -> Sensors/3(In4)
  " Actuators"/2(Out5) -> [LockupCmd]
  "In1 "/1 -> " Actuators"/1(In1)
  Sensors/1(Out1) -> Out1/1
  [TransEstGear] -> Gearbox/1(TransEstGear)
  Torque Converter/1(tc_shaft_out) -> Gearbox/2(gb_trq_in gb_inertia_in)
  GearboxSpdOut/1 -> Gearbox/3(gb_spd_out)
  [LockupCmd] -> Torque Converter/1(tc_lockup)
  [gb_trq_ratio] -> Sensors/7(In1)

== system HybridPowertrain_TestBench_Final/Wheels/Force calculation ==
  spd in : Inport
  BPP[%] : Inport  Port=2
  whl_spd : Inport  Port=3
  grade : Inport  Port=4
  trq_in : Inport  Port=5
  Inertia_In : Inport  Port=6
  "1\\radius " : Gain  Gain=1/whl.plant.init.radius  SaturateOnIntegerOverflow=on  OutDataTypeStr=Inherit: Same as input  ParamDataTypeStr=Inherit: Same as input
  1\radius 1 : Gain  Gain=-1/100  SaturateOnIntegerOverflow=on  OutDataTypeStr=Inherit: Same as input  ParamDataTypeStr=Inherit: Same as input
  Blending : Subsystem  mask(State dependent blending){xl=-0.1, yl=-1, xc=0, yc=0, xr=0.1, yr=1}
      mask prompts: xl "Left point (x-value):"; yl "Left point (y-value):"; xc "Center point (x-value):"; yc "Center point (y-value):"; xr "Right point (x-value):"; yr "Right point (y-vector):"
      mask Display: plot([-1 1 3 6 8], [1.5 1.5 0.5 4.0 4.0])
  Derivative : Derivative
  Divide : Product  Inputs=**
  Rolling Resistance : Subsystem
  Saturation1 : Saturate  UpperLimit=0  LowerLimit=-inf
  Scope : Scope
  Sum2 : Sum  Inputs=++--  SaturateOnIntegerOverflow=on  InputSameDT=on  OutDataTypeStr=Inherit: Same as first input
  Sum6 : Sum  SaturateOnIntegerOverflow=on  InputSameDT=on  OutDataTypeStr=Inherit: Same as first input
  trq_brake_max : Gain  Gain=whl.plant.init.trq_brake_max
  wheel inertia : Constant  Value=whl.plant.init.inertia
  force : Outport
  wires:
  Rolling Resistance/1(rolling resistance) -> Sum2/3
  grade/1 -> Rolling Resistance/2(grade)
  whl_spd/1 -> Rolling Resistance/1(whl_spd)
  trq_brake_max/1 -> Blending/1(input)
  Sum2/1 -> "1\\radius "/1
  Saturation1/1 -> Scope/1, Sum2/1
  BPP[%]/1 -> 1\radius 1/1  "brake cmd"
  spd in/1 -> Derivative/1, Blending/2(Control (state))
  trq_in/1 -> Sum2/2
  1\radius 1/1 -> trq_brake_max/1
  "1\\radius "/1 -> force/1
  Blending/1(Out1) -> Saturation1/1
  Inertia_In/1 -> Sum6/2
  Derivative/1 -> Divide/2
  Divide/1 -> Sum2/4
  wheel inertia/1 -> Sum6/1
  Sum6/1 -> Divide/1

== system HybridPowertrain_TestBench_Final/Wheels/Mass calculation ==
  inertia in : Inport
  1\radius^2 : Gain  Gain=1/whl.plant.init.radius^2  SaturateOnIntegerOverflow=on  OutDataTypeStr=Inherit: Same as input  ParamDataTypeStr=Inherit: Same as input
  Sum6 : Sum  SaturateOnIntegerOverflow=on  InputSameDT=on  OutDataTypeStr=Inherit: Same as first input
  wheel inertia : Constant  Value=whl.plant.init.inertia
  Mass : Outport
  wires:
  inertia in/1 -> Sum6/2
  1\radius^2/1 -> Mass/1
  Sum6/1 -> 1\radius^2/1
  wheel inertia/1 -> Sum6/1

== system HybridPowertrain_TestBench_Final/Wheels/Speed calculation ==
  chas_spd : Inport
  spd in : Outport
  wires:
  chas_spd/1 -> spd in/1

== system HybridPowertrain_TestBench_Final/Differential/Torque calculation/Blending (state dependent) ==
  Input : Inport
  Control (state) : Inport  Port=2
  Linear spline : Fcn  Expr=(u<xl)*yl + (xl<=u)*(u<xc)*((yc-yl)*(u-xl)/(xc-xl)+yl) + (xc<=u)*(u<xr)*((yc-yr)*(u-xr)/(xc-xr)+yr) + (xr<=u)*yr
  Product2 : Product  SaturateOnIntegerOverflow=on  InputSameDT=on  OutDataTypeStr=Inherit: Same as first input
  Output : Outport
  wires:
  Input/1 -> Product2/1
  Linear spline/1 -> Product2/2
  Product2/1 -> Output/1
  Control (state)/1 -> Linear spline/1

== system HybridPowertrain_TestBench_Final/Differential/Torque calculation/Look-Up Table (2-D) ==
  Rows : Inport
  Cols : Inport  Port=2
  Look-Up Table (2-D) : Lookup2D  RowIndex=x  ColumnIndex=y  Table=t  SaturateOnIntegerOverflow=on  InputSameDT=on
  Out1 : Outport
  wires:
  Rows/1 -> Look-Up Table (2-D)/1
  Cols/1 -> Look-Up Table (2-D)/2
  Look-Up Table (2-D)/1 -> Out1/1

== system HybridPowertrain_TestBench_Final/Driver/Driver Control/Override CS SW ==
  note: Override Switch Subsystem
  note: This subsystem is used to override the model value of a signal to a constant value
  In1 : Inport
  Multiport Switch : MultiPortSwitch  DataPortOrder=Zero-based contiguous  Inputs=2  zeroidx=on
  Override Value : Constant  Value=0  OutDataTypeStr=double
  Signal Override Switch 0 = Use Model 1 = Use Constant : Constant
  Out1 : Outport
  wires:
  Override Value/1 -> Multiport Switch/3
  Multiport Switch/1 -> Out1/1
  In1/1 -> Multiport Switch/2
  Signal Override Switch 0 = Use Model 1 = Use Constant/1 -> Multiport Switch/1

== system HybridPowertrain_TestBench_Final/Driver/Driver Control/Override Engine SW ==
  note: This subsystem is used to override the model value of a signal to a constant value
  note: Override Switch Subsystem
  In1 : Inport
  Multiport Switch : MultiPortSwitch  DataPortOrder=Zero-based contiguous  Inputs=2  zeroidx=on
  Override Value : Constant  Value=0  OutDataTypeStr=double
  Signal Override Switch 0 = Use Model 1 = Use Constant : Constant
  Out1 : Outport
  wires:
  Signal Override Switch 0 = Use Model 1 = Use Constant/1 -> Multiport Switch/1
  In1/1 -> Multiport Switch/2
  Multiport Switch/1 -> Out1/1
  Override Value/1 -> Multiport Switch/3

== system HybridPowertrain_TestBench_Final/Driver/Driver Control/Override Regen SW ==
  note: Override Switch Subsystem
  note: This subsystem is used to override the model value of a signal to a constant value
  In1 : Inport
  Multiport Switch : MultiPortSwitch  DataPortOrder=Zero-based contiguous  Inputs=2  zeroidx=on
  Override Value : Constant  Value=0  OutDataTypeStr=double
  Signal Override Switch 0 = Use Model 1 = Use Constant : Constant
  Out1 : Outport
  wires:
  Override Value/1 -> Multiport Switch/3
  Multiport Switch/1 -> Out1/1
  In1/1 -> Multiport Switch/2
  Signal Override Switch 0 = Use Model 1 = Use Constant/1 -> Multiport Switch/1

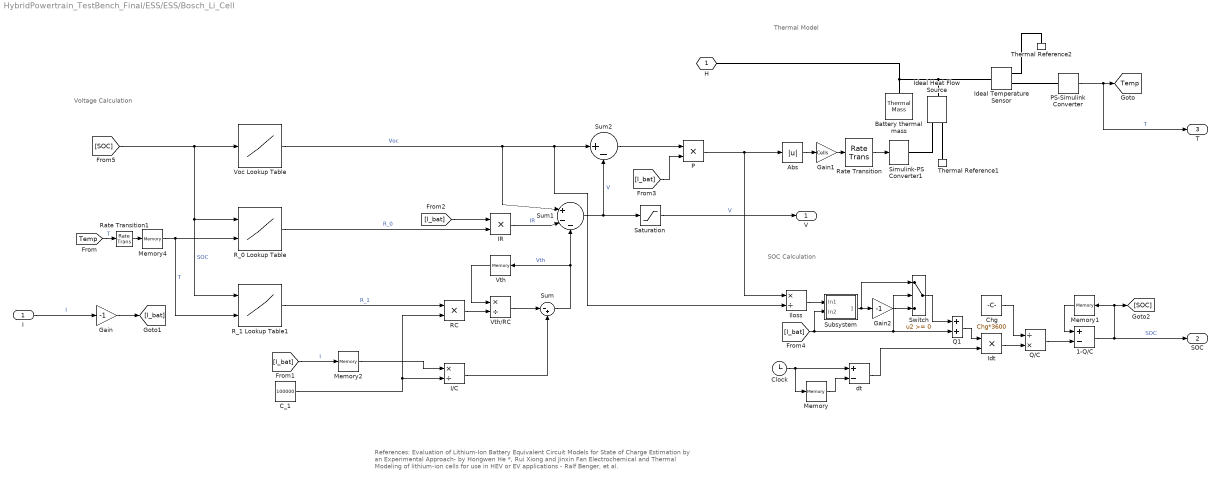
== system HybridPowertrain_TestBench_Final/ESS/ESS/Bosch_Li_Cell ==
  note: References:
      | Evaluation of Lithium-Ion Battery Equivalent Circuit Models for State of Charge Estimation by an Experimental Approach- by Hongwen He *, Rui Xiong and Jinxin Fan
      | Electrochemical and Thermal Modeling of lithium-ion cells for use in HEV or EV applications - Ralf Benger, et al.
  note: Voltage Calculation
  note: Thermal Model
  note: SOC Calculation
  I : Inport
  1-Q/C : Sum  Inputs=+-
  Abs : Abs
  Battery thermal mass : fl_lib/Thermal/Thermal Elements/Thermal Mass  mass=Cells kg  sp_heat=447 J/kg/K  Q_specify=off  Q_priority=High  Q=0 J/s  T_specify=off  T_priority=High  T=300 K
  C_1 : Constant  Value=100000
  Chg : Constant  Value=Chg*3600
  Clock : Clock
  Gain : Gain  Gain=-1
  Gain1 : Gain  Gain=Cells
  Gain2 : Gain  Gain=-1
  I/C : Product  Inputs=*/
  IR : Product  Inputs=**
  Ideal Temperature Sensor : fl_lib/Thermal/Thermal Sensors/Ideal Temperature Sensor
      settings: SourceProductName=Simscape  SourceProductBaseCode=SS
  Ideal Heat Flow Source : fl_lib/Thermal/Thermal Sources/Ideal Heat Flow Source
      settings: SourceProductName=Simscape  SourceProductBaseCode=SS
  Idt : Product  Inputs=**
  Iloss : Product  Inputs=*/
  Memory : Memory  InheritSampleTime=on
  Memory1 : Memory  X0=SOC_init/100  InheritSampleTime=on
  Memory2 : Memory  InheritSampleTime=on
  Memory4 : Memory  X0=298
  P : Product  Inputs=**
  PS-Simulink Converter : nesl_utility/PS-Simulink Converter  PhysicalDomain=network_engine_domain  SubClassName=ps_output  LeftPortType=input  RightPortType=output  PseudoPeriodic=off  Frequencies=[]  Unit=1  AffineConversion=off
  Q/C : Product  Inputs=/*
  Q1 : Sum
  RC : Product  Inputs=**
  R_0 Lookup Table : Lookup_n-D  BreakpointsForDimension1=SOC_bp  BreakpointsForDimension2=T_bp  Table=R_0  InternalRulePriority=Speed  RndMeth=Simplest  InputSameDT=on
  R_1 Lookup Table1 : Lookup_n-D  BreakpointsForDimension1=SOC_bp  BreakpointsForDimension2=T_bp  Table=R_1  InternalRulePriority=Speed  RndMeth=Simplest  InputSameDT=on
  Rate Transition : RateTransition
  Rate Transition1 : RateTransition
  Saturation : Saturate  UpperLimit=4.2  LowerLimit=2.8
  Simulink-PS Converter1 : nesl_utility/Simulink-PS Converter  PhysicalDomain=network_engine_domain  SubClassName=ps_input  LeftPortType=input  RightPortType=output  PseudoPeriodic=off  Frequencies=[]  NoiseDistribution=none  NoiseParameters=[]  Unit=1  AffineConversion=off  InputFiltering=off  SimscapeFilterOrder=1  InputFilterTimeConstant=0.001  UdotUserProvided=1
  Subsystem : Subsystem
  Sum : Sum  Inputs=|-+
  Sum1 : Sum  Inputs=|+--
  Sum2 : Sum  Inputs=|+-
  Switch : Switch
  Thermal Reference1 : fl_lib/Thermal/Thermal Elements/Thermal Reference
  Thermal Reference2 : fl_lib/Thermal/Thermal Elements/Thermal Reference
  Voc Lookup Table : Lookup_n-D  NumberOfTableDimensions=1  BreakpointsForDimension1=SOC_bp  Table=Em  InternalRulePriority=Speed  RndMeth=Simplest  InputSameDT=on
  Vth : Memory  InheritSampleTime=on  LinearizeAsDelay=on
  Vth/RC : Product  Inputs=*/
  dt : Sum  Inputs=+-
  H : PMIOPort  Tag=PMCPort  Port=1  Side=Left
  V : Outport
  SOC : Outport  Port=2
  T : Outport  Port=3
  tag scope: Temp=global
  wires:
  Vth/RC/1 -> Sum/1
  R_0 Lookup Table/1 -> IR/2  "R_0"
  [I_bat] -> Subsystem/2(In2), Q1/2, Switch/2
  Abs/1 -> Gain1/1
  Rate Transition/1 -> Simulink-PS Converter1/1
  [Temp] -> Rate Transition1/1  "T"
  [SOC] -> R_0 Lookup Table/1, R_1 Lookup Table1/1, Voc Lookup Table/1  "SOC"
  IR/1 -> Sum1/2  "IR"
  Sum/1 -> Sum1/3, Vth/1  "Vth"
  Sum2/1 -> P/1
  C_1/1 -> RC/2, I/C/2
  RC/1 -> Vth/RC/2
  [I_bat] -> Memory2/1  "I"
  I/C/1 -> Sum/2
  Vth/1 -> Vth/RC/1
  Sum1/1 -> Saturation/1, Sum2/2  "V"
  [I_bat] -> IR/1
  [I_bat] -> P/2
  PS-Simulink Converter/1 -> T/1, [Temp]  "T"
  R_1 Lookup Table1/1 -> RC/1  "R_1"
  Voc Lookup Table/1 -> Iloss/2, Sum2/1, Sum1/1  "Voc"
  I/1 -> Gain/1  "I"
  Saturation/1 -> V/1  "V"
  Memory4/1 -> R_1 Lookup Table1/2, R_0 Lookup Table/2  "T"
  1-Q/C/1 -> SOC/1, Memory1/1, [SOC]  "SOC"
  Chg/1 -> Q/C/1
  Q/C/1 -> 1-Q/C/2
  Memory1/1 -> 1-Q/C/1
  Gain/1 -> [I_bat]
  Clock/1 -> Memory/1, dt/1
  Memory/1 -> dt/2
  dt/1 -> Idt/2
  Idt/1 -> Q/C/2
  Memory2/1 -> I/C/1
  P/1 -> Iloss/1, Abs/1
  Gain1/1 -> Rate Transition/1
  Gain2/1 -> Switch/3
  Q1/1 -> Idt/1
  Switch/1 -> Q1/1
  Iloss/1 -> Subsystem/1(In1)
  Subsystem/1(Out1) -> Switch/1, Gain2/1
  Rate Transition1/1 -> Memory4/1
  connections:
  Ideal Temperature Sensor/LConn1 -- Ideal Heat Flow Source/LConn1 -- H/RConn1 -- Battery thermal mass/LConn1
  Thermal Reference1/LConn1 -- Ideal Heat Flow Source/RConn2
  Ideal Temperature Sensor/RConn1 -- Thermal Reference2/LConn1
  PS-Simulink Converter/LConn1 -- Ideal Temperature Sensor/RConn2
  Ideal Heat Flow Source/RConn1 -- Simulink-PS Converter1/RConn1

== system HybridPowertrain_TestBench_Final/ESS/ESS/Cooling_Loop ==
  Constant : Constant  Value=Atm_temp+273+0.5
  Convective Heat Transfer : fl_lib/Thermal/Thermal Elements/Convective Heat Transfer  area=1e-4*Cells m^2  heat_tr_coeff=20 W/(m^2 * K)  Q_specify=off  Q_priority=High  Q=0 J/s  T_specify=off  T_priority=High  T=0 K
  Ideal Temperature Source : fl_lib/Thermal/Thermal Sources/Ideal Temperature Source
      settings: SourceProductName=Simscape  SourceProductBaseCode=SS
  Simulink-PS Converter : nesl_utility/Simulink-PS Converter  PhysicalDomain=network_engine_domain  SubClassName=ps_input  LeftPortType=input  RightPortType=output  PseudoPeriodic=off  Frequencies=[]  NoiseDistribution=none  NoiseParameters=[]  Unit=1  AffineConversion=off  InputFiltering=off  SimscapeFilterOrder=1  InputFilterTimeConstant=0.001  UdotUserProvided=1
  Solver Configuration : nesl_utility/Solver Configuration  PhysicalDomain=network_engine_domain  SubClassName=solver  LeftPortType=input  RightPortType=generic  Accelerate=off  Tones=[]  Harmonics=[]  SimulateNoise=off  Profile=off  UseLocalSampling=off  EnableSwitchedLinearOptims=on  FrequencyDomain=off  UseCCode=off  RelTol=0.001  AbsTol=1e-06  MinStep=1e-09  ToWorkspace=off  RevertToSquareIcSolve=off  NumHomotopyIterations=100  DoDC=off  ResidualTolerance=1e-09  UseLocalSolver=off  LocalSolverChoice=NE_BACKWARD_EULER_ADVANCER  LocalSolverSampleTime=0.001  DoFixedCost=off  MaxNonlinIter=3  MaxModeIter=2  LinearAlgebra=Sparse  DelaysMemoryBudget=1024  AutomaticFiltering=on  FilteringTimeConstant=0.001
  Thermal Reference : fl_lib/Thermal/Thermal Elements/Thermal Reference
  Conn1 : PMIOPort  Port=1  Side=Right
  wires:
  Constant/1 -> Simulink-PS Converter/1
  connections:
  Thermal Reference/LConn1 -- Ideal Temperature Source/RConn2
  Ideal Temperature Source/LConn1 -- Convective Heat Transfer/RConn1
  Simulink-PS Converter/RConn1 -- Ideal Temperature Source/RConn1
  Convective Heat Transfer/LConn1 -- Solver Configuration/RConn1 -- Conn1/RConn1

== system HybridPowertrain_TestBench_Final/ESS/ESS/Cooling_Loop1 ==
  ACcompRPM : Constant  Value=8600
  Add : Sum  Inputs=--
  Add2 : Sum  Inputs=+-
  Add4 : Sum  Inputs=+-
  Constant3 : Constant  Value=0
  CoolaSpecHeat : Constant  Value=4200
  Divide{4..6,8} (4 alike) : Product  Inputs=**
  Gain : Gain  Gain=1/1000
  Gain1 : Gain  Gain=1/6000
  Ideal Heat Flow Sensor : fl_lib/Thermal/Thermal Sensors/Ideal Heat Flow Sensor
      settings: SourceProductName=Simscape  SourceProductBaseCode=SS
  Ideal Heat Flow Source : fl_lib/Thermal/Thermal Sources/Ideal Heat Flow Source
      settings: SourceProductName=Simscape  SourceProductBaseCode=SS
  K : Constant  Value=273.15
  PS-Simulink Converter : nesl_utility/PS-Simulink Converter  PhysicalDomain=network_engine_domain  SubClassName=ps_output  LeftPortType=input  RightPortType=output  PseudoPeriodic=off  Frequencies=[]  Unit=1  AffineConversion=off
  PumpFlowRate : Constant  Value=1.8
  Rate Transition1 : RateTransition
  Scope : Scope
  Sensor : Subsystem
  Simulink-PS Converter3 : nesl_utility/Simulink-PS Converter  PhysicalDomain=network_engine_domain  SubClassName=ps_input  LeftPortType=input  RightPortType=output  PseudoPeriodic=off  Frequencies=[]  NoiseDistribution=none  NoiseParameters=[]  Unit=1  AffineConversion=off  InputFiltering=off  SimscapeFilterOrder=1  InputFilterTimeConstant=0.001  UdotUserProvided=1
  Solver Configuration1 : nesl_utility/Solver Configuration  PhysicalDomain=network_engine_domain  SubClassName=solver  LeftPortType=input  RightPortType=generic  Accelerate=off  Tones=[]  Harmonics=[]  SimulateNoise=off  Profile=off  UseLocalSampling=off  EnableSwitchedLinearOptims=on  FrequencyDomain=off  UseCCode=off  RelTol=0.001  AbsTol=1e-06  MinStep=1e-09  ToWorkspace=off  RevertToSquareIcSolve=off  NumHomotopyIterations=100  DoDC=off  ResidualTolerance=1e-09  UseLocalSolver=off  LocalSolverChoice=NE_BACKWARD_EULER_ADVANCER  LocalSolverSampleTime=0.001  DoFixedCost=off  MaxNonlinIter=3  MaxModeIter=2  LinearAlgebra=Sparse  DelaysMemoryBudget=1024  AutomaticFiltering=on  FilteringTimeConstant=0.001
  Switch : Switch  Criteria=u2 ~= 0
  Thermal Reference3 : fl_lib/Thermal/Thermal Elements/Thermal Reference
  coolant_temp : Constant  Value=25
  h : Gain  Gain=1000/3600
  tloop : Gain  Gain=0.01
  Conn2 : PMIOPort  Port=1  Side=Left
  wires:
  [ESSCompEna] -> Switch/2
  Divide6/1 -> Divide4/2
  tloop/1 -> Divide6/2
  Divide8/1 -> Gain/1
  Add4/1 -> Divide4/1
  CoolaSpecHeat/1 -> Divide6/1
  coolant_temp/1 -> Add4/2
  h/1 -> Divide5/2
  Gain/1 -> Gain1/1  "1/kw"
  [ACComp_control] -> Switch/1
  Gain1/1 -> Add/1  "r/min"
  ACcompRPM/1 -> Divide8/2
  Divide5/1 -> tloop/1
  PumpFlowRate/1 -> h/1  "m^3/h"
  Divide4/1 -> Add/2
  Constant3/1 -> Switch/3
  Add2/1 -> Add4/1
  [ess_temp] -> Add2/1
  K/1 -> Add2/2
  Rate Transition1/1 -> Simulink-PS Converter3/1
  Add/1 -> Rate Transition1/1
  Switch/1 -> Divide8/1
  [ESS_pump_control] -> Divide5/1
  PS-Simulink Converter/1 -> Scope/1
  connections:
  Ideal Heat Flow Source/LConn1 -- Ideal Heat Flow Sensor/LConn1 -- Sensor/LConn1
  Simulink-PS Converter3/RConn1 -- Ideal Heat Flow Source/RConn1
  Thermal Reference3/LConn1 -- Ideal Heat Flow Source/RConn2
  Solver Configuration1/RConn1 -- Ideal Heat Flow Sensor/RConn2 -- Conn2/RConn1
  Ideal Heat Flow Sensor/RConn1 -- PS-Simulink Converter/LConn1

== system HybridPowertrain_TestBench_Final/ESS/ESS/Fault_Insertion ==
  In1 : Inport
  Gain : Gain  Gain=3
  Switch : Switch  Threshold=1
  Out1 : Outport
  wires:
  [ESSOverTemp] -> Switch/2
  In1/1 -> Gain/1, Switch/3
  Switch/1 -> Out1/1  "temp"
  Gain/1 -> Switch/1

== system HybridPowertrain_TestBench_Final/ESS/Inputs/CAN_fromHCU ==
  Bus Creator : BusCreator  Inputs=2
  Outputs : Outport
  wires:
  [HCU_to_HV_CAN] -> Bus Creator/1
  [HCU_to_EBCAN] -> Bus Creator/2
  Bus Creator/1 -> Outputs/1

== system HybridPowertrain_TestBench_Final/ESS/Inputs/Digital_fromHCU ==
  Outputs : Outport
  wires:
  [Digital] -> Outputs/1

== system HybridPowertrain_TestBench_Final/ESS/Soft BMS/BMS_08 1 ==
  Bus Creator8 : BusCreator  Inputs=9
  BMS_08 : Outport
  wires:
  [BMS_Temp_Zelle_Min] -> Bus Creator8/2  "BMS_Temp_Zelle_Min"
  Bus Creator8/1 -> BMS_08/1  "BMS_08"
  ? -> Bus Creator8/8
  ? -> Bus Creator8/6
  ? -> Bus Creator8/4
  ? -> Bus Creator8/3
  [BMS_Temp_Zelle_Max] -> Bus Creator8/1  "BMS_Temp_Zelle_Max"
  ? -> Bus Creator8/7
  ? -> Bus Creator8/9
  ? -> Bus Creator8/5
